simulink model "lab6"  (R2021b)
settings: Solver=ode5  StartTime=0.0  StopTime=100.0  FixedStep=0.01  RelTol=1e-3
undefined symbols (not defined in the file): A, B, C, c1, c2, F1, F2, k, L, s
settings Model: Creator=Student  LastModifiedBy=Marcin

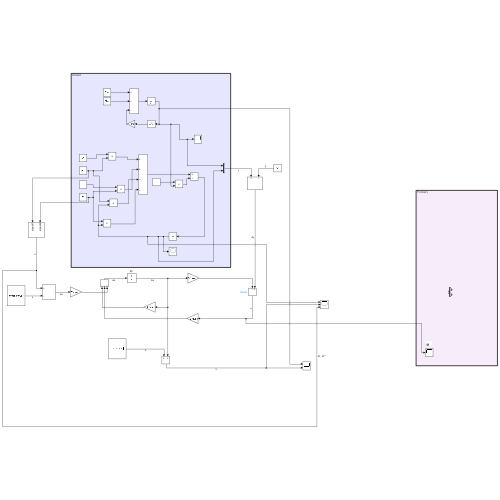
[thumbnail: Simulink's stored preview of the top-level diagram]
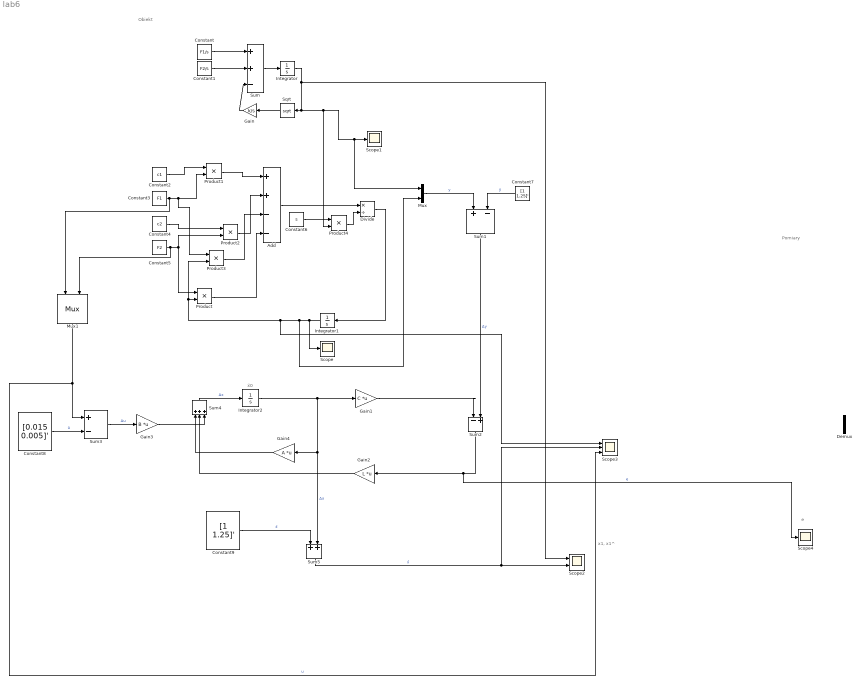
== system lab6 ==
  note: e
  note: Pomiary
  note: x̂0
  note: Obiekt
  note: x1, x1^
  Add : Sum  Inputs=++--
  Constant : Constant  Value=F1/s
  Constant1 : Constant  Value=F2/s
  Constant2 : Constant  Value=c1
  Constant3 : Constant  Value=F1
  Constant4 : Constant  Value=c2
  Constant5 : Constant  Value=F2
  Constant6 : Constant  Value=s
  Constant7 : Constant  Value=[1 1.25]'
  Constant8 : Constant  Value=[0.015 0.005]'
  Constant9 : Constant  Value=[1 1.25]'
  Demux : Demux  Outputs=2
  Divide : Product  Inputs=*/
  Gain : Gain  Gain=k/s
  Gain1 : Gain  Gain=C  Multiplication=Matrix(K*u) (u vector)
  Gain2 : Gain  Gain=L  Multiplication=Matrix(K*u) (u vector)
  Gain3 : Gain  Gain=B  Multiplication=Matrix(K*u) (u vector)
  Gain4 : Gain  Gain=A  Multiplication=Matrix(K*u) (u vector)
  Integrator : Integrator  InitialCondition=1
  Integrator1 : Integrator  InitialCondition=1.25
  Integrator2 : Integrator  InitialCondition=[0.01 0.1]'
  Mux : Mux  Inputs=2
  Mux1 : Mux  Inputs=2
      settings: DisplayOption=signals
  Product{,1..4} (5 alike) : Product
  Scope : Scope
  Scope1 : Scope
  Scope2 : Scope  NumInputPorts=2
  Scope3 : Scope  NumInputPorts=3
  Scope4 : Scope
  Sqrt : Sqrt  SaturateOnIntegerOverflow=on
  Sum : Sum  Inputs=++-
  Sum1 : Sum  Inputs=+-
  Sum2 : Sum  Inputs=|-+
  Sum3 : Sum  Inputs=+-
  Sum4 : Sum  Inputs=+++
  Sum5 : Sum
  wires:
  Constant/1 -> Sum/1
  Constant1/1 -> Sum/2
  Sum/1 -> Integrator/1
  Integrator/1 -> Scope2/1, Mux/1, Scope1/1, Product4/2, Sqrt/1
  Sqrt/1 -> Gain/1
  Gain/1 -> Sum/3
  Constant2/1 -> Product1/1
  Constant3/1 -> Product3/1, Product1/2, Mux1/1
  Constant4/1 -> Product2/1
  Constant5/1 -> Product/1, Product2/2, Mux1/2
  Product1/1 -> Add/1
  Product2/1 -> Add/2
  Product3/1 -> Add/3
  Product/1 -> Add/4
  Add/1 -> Divide/1
  Constant6/1 -> Product4/1
  Product4/1 -> Divide/2
  Divide/1 -> Integrator1/1
  Mux/1 -> Sum1/1  "y"
  Sum1/1 -> Sum2/2  "Δy"
  Constant7/1 -> Sum1/2  "ȳ"
  Gain1/1 -> Sum2/1
  Sum2/1 -> Scope4/1, Gain2/1  "e"
  Gain2/1 -> Sum4/2
  Sum4/1 -> Integrator2/1  "Δx"
  Integrator2/1 -> Gain4/1, Sum5/2, Gain1/1  "Δẋ"
  Gain3/1 -> Sum4/3
  Gain4/1 -> Sum4/1
  Mux1/1 -> Scope3/3, Sum3/1  "u"
  Sum3/1 -> Gain3/1  "Δu"
  Constant8/1 -> Sum3/2  "ū"
  Constant9/1 -> Sum5/1  "x̄"
  Sum5/1 -> Scope2/2, Scope3/2  "x̂"
  Integrator1/1 -> Scope/1, Mux/2, Scope3/1, Product3/2, Product/2
